simulink model "KneeReflexDemo"  (R2025b)
settings: Solver=ode45  StartTime=0.0  StopTime=5  RelTol=1e-3
PreLoadFcn:
  | I_knee = 0.06;      % kg*m^2 below-knee inertia (rig estimate)
  | b_knee = 0.5;        % N*m*s/rad joint damping
  | K_knee = 0.5;       % N*m/rad return spring
  | th0    = 0.26;      % rad spring rest angle (~15 deg)
  | ROM    = 1.5708;    % rad (90 deg) normalizing range
  | r_arm  = 0.035;     % m BPA moment arm
  | Tload  = 0.5;       % N*m constant flexion load torque
  | desc_ext = 4.2;     % nA descending drive to extensor MN
  | desc_flex = 2.5;    % nA descending drive to flexor MN
  | Fmax_ext = 500;     % N
  | Fmax_flex = 450;    % N
  | epsScale = 0.15;    % muscle strain span over full joint ROM
libraries: SNS_Library x20
settings Model: Creator=Ben  LastModifiedBy=Ben

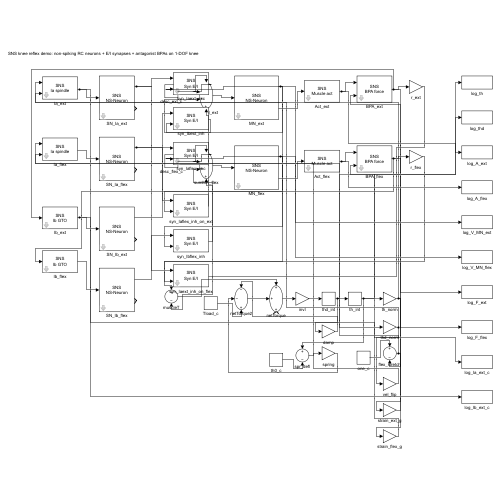
[thumbnail: Simulink's stored preview of the top-level diagram]
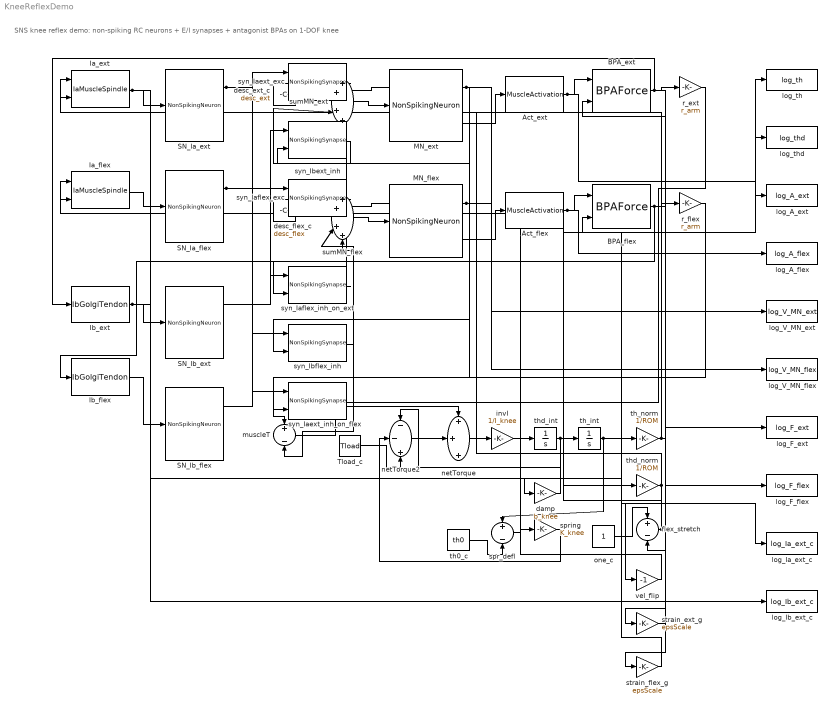
== system KneeReflexDemo ==
  note: SNS knee reflex demo: non-spiking RC neurons + E/I synapses + antagonist BPAs on 1-DOF knee
  Act_ext : SNS_Library/MuscleActivation  tauAct=50
  Act_flex : SNS_Library/MuscleActivation  tauAct=50
  BPA_ext : SNS_Library/BPAForce  Fmax=Fmax_ext  epsMax=0.25
  BPA_flex : SNS_Library/BPAForce  Fmax=Fmax_flex  epsMax=0.25
  Ia_ext : SNS_Library/IaMuscleSpindle  Imax=10  Wl=6  Wv=8
  Ia_flex : SNS_Library/IaMuscleSpindle  Imax=10  Wl=6  Wv=8
  Ib_ext : SNS_Library/IbGolgiTendon  Imax=10  Kf=0.02
  Ib_flex : SNS_Library/IbGolgiTendon  Imax=10  Kf=0.0222
  MN_ext : SNS_Library/NonSpikingNeuron  Vrest=-52  Gm=0.5  Cm=2.5  Thr=-45  Slope=1
  MN_flex : SNS_Library/NonSpikingNeuron  Vrest=-52  Gm=0.5  Cm=2.5  Thr=-45  Slope=1
  SN_Ia_ext : SNS_Library/NonSpikingNeuron  Vrest=-52  Gm=0.4  Cm=2  Thr=-55  Slope=1
  SN_Ia_flex : SNS_Library/NonSpikingNeuron  Vrest=-52  Gm=0.4  Cm=2  Thr=-55  Slope=1
  SN_Ib_ext : SNS_Library/NonSpikingNeuron  Vrest=-52  Gm=0.4  Cm=2  Thr=-55  Slope=1
  SN_Ib_flex : SNS_Library/NonSpikingNeuron  Vrest=-52  Gm=0.4  Cm=2  Thr=-55  Slope=1
  Tload_c : Constant  Value=Tload
  damp : Gain  Gain=b_knee
  desc_ext_c : Constant  Value=desc_ext
  desc_flex_c : Constant  Value=desc_flex
  flex_stretch : Sum  Inputs=+-
  invI : Gain  Gain=1/I_knee
  log_A_ext : ToWorkspace  VariableName=log_A_ext  SaveFormat=Timeseries  SampleTime=-1
  log_A_flex : ToWorkspace  VariableName=log_A_flex  SaveFormat=Timeseries  SampleTime=-1
  log_F_ext : ToWorkspace  VariableName=log_F_ext  SaveFormat=Timeseries  SampleTime=-1
  log_F_flex : ToWorkspace  VariableName=log_F_flex  SaveFormat=Timeseries  SampleTime=-1
  log_Ia_ext_c : ToWorkspace  VariableName=log_Ia_ext_c  SaveFormat=Timeseries  SampleTime=-1
  log_Ib_ext_c : ToWorkspace  VariableName=log_Ib_ext_c  SaveFormat=Timeseries  SampleTime=-1
  log_V_MN_ext : ToWorkspace  VariableName=log_V_MN_ext  SaveFormat=Timeseries  SampleTime=-1
  log_V_MN_flex : ToWorkspace  VariableName=log_V_MN_flex  SaveFormat=Timeseries  SampleTime=-1
  log_th : ToWorkspace  VariableName=log_th  SaveFormat=Timeseries  SampleTime=-1
  log_thd : ToWorkspace  VariableName=log_thd  SaveFormat=Timeseries  SampleTime=-1
  muscleT : Sum  Inputs=+-
  netTorque : Sum  Inputs=+++
  netTorque2 : Sum  Inputs=--+
  one_c : Constant
  r_ext : Gain  Gain=r_arm
  r_flex : Gain  Gain=r_arm
  spr_defl : Sum  Inputs=+-
  spring : Gain  Gain=K_knee
  strain_ext_g : Gain  Gain=epsScale
  strain_flex_g : Gain  Gain=epsScale
  sumMN_ext : Sum  Inputs=++++
  sumMN_flex : Sum  Inputs=++++
  syn_Iaext_exc : SNS_Library/NonSpikingSynapse  gmax=0.18  Esyn=0  ThrPre=-45  SlopePre=0.5
  syn_Iaext_inh_on_flex : SNS_Library/NonSpikingSynapse  gmax=0.15  Esyn=-72  ThrPre=-45  SlopePre=0.5
  syn_Iaflex_exc : SNS_Library/NonSpikingSynapse  gmax=0.18  Esyn=0  ThrPre=-45  SlopePre=0.5
  syn_Iaflex_inh_on_ext : SNS_Library/NonSpikingSynapse  gmax=0.15  Esyn=-72  ThrPre=-45  SlopePre=0.5
  syn_Ibext_inh : SNS_Library/NonSpikingSynapse  gmax=0.20  Esyn=-72  ThrPre=-45  SlopePre=0.5
  syn_Ibflex_inh : SNS_Library/NonSpikingSynapse  gmax=0.20  Esyn=-72  ThrPre=-45  SlopePre=0.5
  th0_c : Constant  Value=th0
  th_int : Integrator  InitialCondition=0.26
  th_norm : Gain  Gain=1/ROM
  thd_int : Integrator
  thd_norm : Gain  Gain=1/ROM
  vel_flip : Gain  Gain=-1
  wires:
  netTorque/1 -> invI/1
  invI/1 -> thd_int/1
  thd_int/1 -> th_int/1, damp/1, thd_norm/1, log_thd/1
  th_int/1 -> spr_defl/1, th_norm/1, log_th/1
  th0_c/1 -> spr_defl/2
  spr_defl/1 -> spring/1
  muscleT/1 -> netTorque/1
  netTorque2/1 -> netTorque/2
  damp/1 -> netTorque2/1
  spring/1 -> netTorque2/2
  Tload_c/1 -> netTorque2/3
  one_c/1 -> flex_stretch/1
  th_norm/1 -> flex_stretch/2, strain_ext_g/1, Ia_ext/1
  thd_norm/1 -> vel_flip/1, Ia_ext/2
  flex_stretch/1 -> strain_flex_g/1, Ia_flex/1
  vel_flip/1 -> Ia_flex/2
  Ia_ext/1 -> SN_Ia_ext/1, log_Ia_ext_c/1
  Ia_flex/1 -> SN_Ia_flex/1
  Ib_ext/1 -> SN_Ib_ext/1, log_Ib_ext_c/1
  Ib_flex/1 -> SN_Ib_flex/1
  desc_ext_c/1 -> sumMN_ext/1
  desc_flex_c/1 -> sumMN_flex/1
  sumMN_ext/1 -> MN_ext/1
  sumMN_flex/1 -> MN_flex/1
  SN_Ia_ext/1 -> syn_Iaext_exc/1, syn_Iaext_inh_on_flex/1
  SN_Ib_ext/1 -> syn_Ibext_inh/1
  SN_Ia_flex/1 -> syn_Iaflex_inh_on_ext/1, syn_Iaflex_exc/1
  SN_Ib_flex/1 -> syn_Ibflex_inh/1
  MN_ext/1 -> syn_Iaext_exc/2, syn_Ibext_inh/2, syn_Iaflex_inh_on_ext/2, log_V_MN_ext/1
  MN_flex/1 -> syn_Iaflex_exc/2, syn_Ibflex_inh/2, syn_Iaext_inh_on_flex/2, log_V_MN_flex/1
  syn_Iaext_exc/1 -> sumMN_ext/2
  syn_Ibext_inh/1 -> sumMN_ext/3
  syn_Iaflex_inh_on_ext/1 -> sumMN_ext/4
  syn_Iaflex_exc/1 -> sumMN_flex/2
  syn_Ibflex_inh/1 -> sumMN_flex/3
  syn_Iaext_inh_on_flex/1 -> sumMN_flex/4
  MN_ext/2 -> Act_ext/1
  MN_flex/2 -> Act_flex/1
  Act_ext/1 -> BPA_ext/1, log_A_ext/1
  Act_flex/1 -> BPA_flex/1, log_A_flex/1
  strain_ext_g/1 -> BPA_ext/2
  strain_flex_g/1 -> BPA_flex/2
  BPA_ext/1 -> Ib_ext/1, r_ext/1, log_F_ext/1
  BPA_flex/1 -> Ib_flex/1, r_flex/1, log_F_flex/1
  r_flex/1 -> muscleT/1
  r_ext/1 -> muscleT/2
